simulink model "jackfinalAAI"  (R2020a)
settings: Solver=FixedStepAuto  StartTime=0.0  StopTime=10.0  FixedStep=1e-3  RelTol=1e-3  EnableMultiTasking=on
undefined symbols (not defined in the file): D0, D10, D11, D13, D2, D3, D4, D5, D6, D8, PTA0, PTA1, PTA2, PTB23, PTB9, PTC16, PTC2, PTD0, PTD1, PTD2
libraries: frdmk64flib x10
settings Model: ExtModeTrigDuration=5  Creator=jamescameron  LastModifiedBy=jamescameron
settings OptimizationCC: EnhancedBackFolding=on  PassReuseOutputArgsAs=Individual arguments  ZeroExternalMemoryAtStartup=off  ZeroInternalMemoryAtStartup=off  MaxStackSize=64  OptimizeBlockOrder=speed  DifferentSizesBufferReuse=on  OptimizationCustomize=off  EfficientTunableParamExpr=on
settings DebuggingCC: ParameterTunabilityLossMsg=error
settings HardwareCC: ProdBitPerPointer=32  ProdBitPerSizeT=32  ProdBitPerPtrDiffT=32  ProdLargestAtomicInteger=Long  ProdLargestAtomicFloat=Double  ProdWordSize=32  ProdHWDeviceType=ARM Compatible->ARM Cortex
settings SFSimCC: MATLABDynamicMemAlloc=off
settings RTWCC: SystemTargetFile=ert.tlc  HardwareBoard=NXP FRDM-K64F  TemplateMakefile=ert_default_tmf  Toolchain=GNU Tools for ARM Embedded Processors
settings CodeAppCC: ForceParamTrailComments=on  IgnoreCustomStorageClasses=off  OperatorAnnotations=on  SimulinkDataObjDesc=on  SFDataObjDesc=on  InsertBlockDesc=on

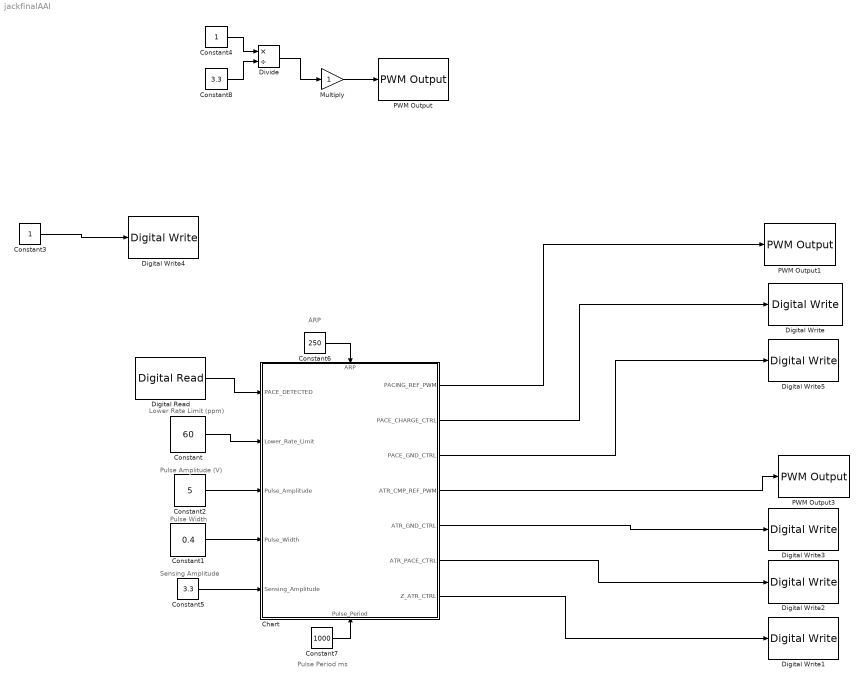
== system jackfinalAAI ==
  note: Pulse Period ms
  note: ARP
  note: Sensing Amplitude
  note: Pulse Amplitude (V)
  note: Lower Rate Limit (ppm)
  note: Pulse Width
  Chart : Stateflow chart  TreatAsAtomicUnit=on
      settings: PortSchema="{\"entries\":[{\"content\":{\"sides\":[{\"content\":{\"connectorIds\":[\"In4\",\"In5\",\"In6\",\"In7\",\"In3\"]},\"type\":\"ConnectorPlacement.EquallySpacedRectSide\",\"uuid\":\"72652cfb-0bb6-4258-a704-601e3c0b5d26\"},{\"content\":{\"connectorIds\":[\"Out1\",\"Out2\",\"Out3\",\"Out4\",\"Out5\",\"Out6\",\"Out7\"],\"side\":\"RIGHT\"},\"type\":\"ConnectorPlacement.EquallySpacedRectSide\",\"uuid\":\"51bd22d5-4d54-4764-997b-ab789807979b\"},{\"content\":{\"connectorIds\":[\"In1\"],\"side\":\"TOP\"},\"type\":\"ConnectorPlacement.EquallySpacedRectSide\",\"uuid\":\"b568f89c-a11f-4812-8dfe-f819792306b3\"},{\"content\":{\"connectorIds\":[\"In2\"],\"side\":\"BOTTOM\"},\"type\":\"ConnectorPlacement.EquallySpacedRectSide\",\"uuid\":\"a4e10e65-0031-4f7f-a850-f9aac3c2f857\"}]},\"type\":\"ConnectorPlacement.EquallySpacedConnector\",\"uuid\":\"bf9daf3b-2142-41fe-accd-96c7a2256776\"}],\"packageUris\":[\"http://schema.mathworks.com/mf0/Connector/19700101\"],\"version\":\"1.0\"}"
  Constant : Constant  Value=60
  Constant1 : Constant  Value=0.4
  Constant2 : Constant  Value=5
  Constant3 : Constant
  Constant4 : Constant
  Constant5 : Constant  Value=3.3
  Constant6 : Constant  Value=250
  Constant7 : Constant  Value=1000
  Constant8 : Constant  Value=3.3
  Digital Read : frdmk64flib/Digital Read  Whichpin=PTC16 (D0)  SampleTime=-1
  Digital Write : frdmk64flib/Digital Write  Whichpin=PTB9 (D2)
  Digital Write1 : frdmk64flib/Digital Write  Whichpin=PTB23 (D4)
  Digital Write2 : frdmk64flib/Digital Write  Whichpin=PTA0 (D8)
  Digital Write3 : frdmk64flib/Digital Write  Whichpin=PTD2 (D11)
  Digital Write4 : frdmk64flib/Digital Write  Whichpin=PTD1 (D13)
  Digital Write5 : frdmk64flib/Digital Write  Whichpin=PTD0 (D10)
  Divide : Product  Inputs=*/
  Multiply : Gain
  PWM Output : frdmk64flib/PWM Output  Whichpin=PTA1 (D3)  InitialFrequency=2000  InitialDutyCycle=0
  PWM Output1 : frdmk64flib/PWM Output  Whichpin=PTA2 (D5)  InitialFrequency=2000  InitialDutyCycle=0
  PWM Output3 : frdmk64flib/PWM Output  Whichpin=PTC2 (D6)  InitialFrequency=2000  InitialDutyCycle=0
  wires:
  Chart/7(Z_ATR_CTRL) -> Digital Write1/1
  Constant6/1 -> Chart/1(ARP)
  Constant5/1 -> Chart/3(Sensing_Amplitude)
  Constant7/1 -> Chart/2(Pulse_Period)
  Chart/4(ATR_CMP_REF_PWM) -> PWM Output3/1
  Constant1/1 -> Chart/7(Pulse_Width)
  Chart/5(ATR_GND_CTRL) -> Digital Write3/1
  Chart/3(PACE_GND_CTRL) -> Digital Write5/1
  Chart/1(PACING_REF_PWM) -> PWM Output1/1
  Constant/1 -> Chart/5(Lower_Rate_Limit)
  Chart/6(ATR_PACE_CTRL) -> Digital Write2/1
  Constant2/1 -> Chart/6(Pulse_Amplitude)
  Chart/2(PACE_CHARGE_CTRL) -> Digital Write/1
  Digital Read/1 -> Chart/4(PACE_DETECTED)
  Constant3/1 -> Digital Write4/1
  Multiply/1 -> PWM Output/1
  Divide/1 -> Multiply/1
  Constant4/1 -> Divide/1
  Constant8/1 -> Divide/2

== stateflow chart jackfinalAAI/Chart ==
  state CHARGING
    entry:
    %%Charging C22
    PACING_REF_PWM = (Pulse_Amplitude/5.0)*100;
    ATR_CMP_REF_PWM = (Sensing_Amplitude/5)*100;
    ATR_PACE_CTRL = 0;
    PACE_CHARGE_CTRL = 1;
    %%Discharging Blocking Cap
    PACE_GND_CTRL = 1;
    Z_ATR_CTRL = 0;
    ATR_GND_CTRL = 1;
  state PACING
    entry:
    PACE_CHARGE_CTRL = 0;
    PACING_REF_PWM = (Pulse_Amplitude/5.0)*100;
    PACE_GND_CTRL = 1;
    Z_ATR_CTRL = 0;
    ATR_GND_CTRL = 0;
    ATR_PACE_CTRL = 1;
  state sense
    entry:
    %%Charging C22
    PACING_REF_PWM = (Pulse_Amplitude/5.0)*100;
    ATR_CMP_REF_PWM = (Sensing_Amplitude/5)*100;
    ATR_PACE_CTRL = 0;
    PACE_CHARGE_CTRL = 1;
    %%Discharging Blocking Cap
    PACE_GND_CTRL = 1;
    Z_ATR_CTRL = 0;
    ATR_GND_CTRL = 1;
  (default) -> CHARGING
  CHARGING -> PACING [order 2] : after(Pulse_Period- Pulse_Width - ARP,msec)[PACE_DETECTED == 0]
  CHARGING -> sense [order 1] : [PACE_DETECTED == 1]
  sense -> CHARGING : [after(ARP, msec)]
  PACING -> sense : [after(Pulse_Width,msec)]
  data: ARP input; Pulse_Period input; Sensing_Amplitude input; PACE_DETECTED input; PACING_REF_PWM output; PACE_CHARGE_CTRL output; PACE_GND_CTRL output; Lower_Rate_Limit input; Pulse_Amplitude input; Pulse_Width input; ATR_CMP_REF_PWM output; ATR_GND_CTRL output; ATR_PACE_CTRL output; Z_ATR_CTRL output
